simulink model "S2"  (R2025a)
settings: Solver=VariableStepAuto  StartTime=0.0  StopTime=10.0  RelTol=1e-3
settings Model: Creator=a.diteodoro  LastModifiedBy=a.diteodoro

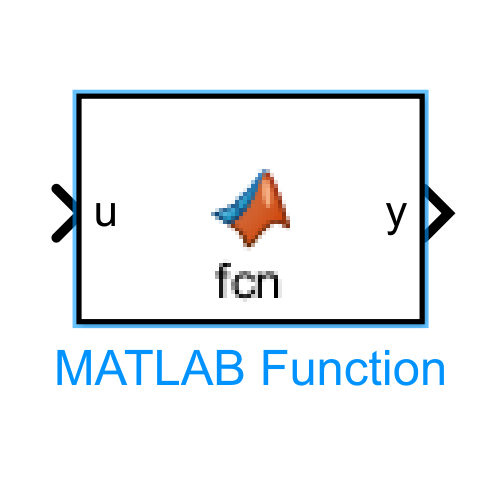
[thumbnail: Simulink's stored preview of the top-level diagram]
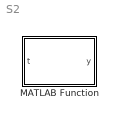
== system S2 ==
  MATLAB Function : MATLAB Function  TreatAsAtomicUnit=on

== matlab function S2/MATLAB Function ==
  data: t input; y output
function y = fcn(t)
y = sin(t);   % puedes cambiarla
end
